simulink library "MarineRoboticsLib"  (R2022b)
settings: Solver=VariableStepAuto  StartTime=0.0  StopTime=10.0  RelTol=1e-3
undefined symbols (not defined in the file): t200_force_n, t200_pwm_n
libraries: $bdroot x13, ros2lib x4, robotcorelib x1
settings Model: Creator=dnad  LastModifiedBy=dnad

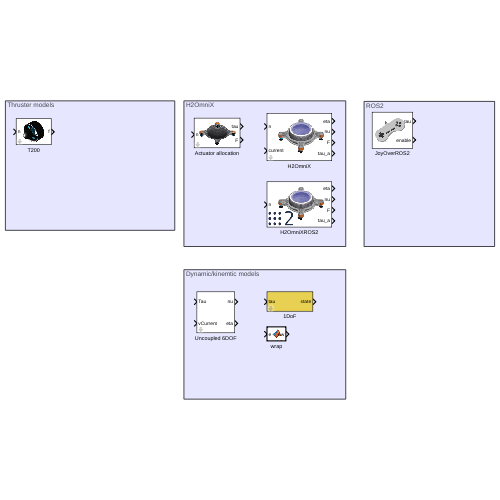
[thumbnail: Simulink's stored preview of the top-level diagram]
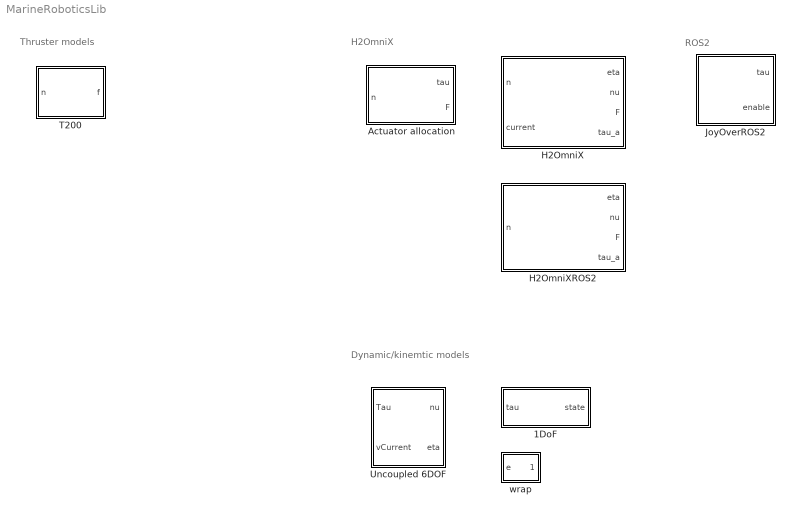
== system MarineRoboticsLib ==
  note: ROS2
  note: Dynamic/kinemtic models
  note: H2OmniX
  note: Thruster models
  1DoF : Subsystem  mask{nu0=0, alpha=0, beta=0, betaa=0}
      mask prompts: nu0 "Initial velocity"; alpha "Intertia"; beta "Linear drag"; betaa "Quadratic drag"
  Actuator allocation : Subsystem  mask(H2OmniX allocation){Tm=0, B=[0.25, 0.25, -0.25, -0.25; -0.25,  0.25, -0.25,  0.25; -0.25, 0.25, 0.25, -0.25], Keff=[1,1,1,1]}
      mask prompts: Tm "ESC time constant"; B "Thruster configuration (allocation) matrix"; Keff "Thruster efficiency (1x4 matrix)"
      mask help: The block perform normalized allocation based on thruster PWM signals and outputs the achieved generalized force and torque (tau).
      mask Display: image('$imagefile'); % Use "Edit Image" on toolstrip to change.
  H2OmniX : Subsystem  mask(H2OmniX){alpha=[2.1,2.1,0.4], beta=[0,0,0.24], betaa=[1,1,0], nu0=[0,0,0], eta0=[0,0,0]}
      mask prompts: alpha "Inertial components"; beta "Linear drag"; betaa "Quadratic drag"; nu0 "Velocities"; eta0 "Position"
      mask help: This block incorporates the H2OmniX model. It takes as input the PWM inputs for individual thrusters and sea current disturbance. It outputs the current velocity and position. For introspective purposes the individual forces applied by each thruster are output as well.
      settings: MinAlgLoopOccurrences=on
      mask DialogControl ParameterGroupVar Prompt: Dynamics
      mask DialogControl Container3 Prompt: Initial state
      mask Display: image('$imagefile'); % Use "Edit Image" on toolstrip to change.
  H2OmniXROS2 : Subsystem
      mask Display: image('$imagefile'); % Use "Edit Image" on toolstrip to change.
  JoyOverROS2 : Subsystem
      mask Display: image('$imagefile'); % Use "Edit Image" on toolstrip to change.
  T200 : Subsystem  mask(T200){Keff=1, Tm=0}
      mask prompts: Keff "Efficiency"; Tm "ESC time constant (Tm)"
      mask help: This simulink block simulates a Blue Robotics T200 thruster on 14V controlled input. The efficiancy parameter given from [0,1] additionally decreases the force output of the thruster. The ESC reaction time is the time constant of the PT1 element included in the model. Put the time constant to zero to have instantaneous response.
      mask Display: image('$imagefile'); % Use "Edit Image" on toolstrip to change.
  Uncoupled 6DOF : Subsystem  mask{nu0=[0,0,0,0,0,0], eta0=[0,0,0,0,0,0], alpha=[0,0,0,0,0,0], beta=[0,0,0,0,0,0], betaa=[0,0,0,0,0,0]}
      mask prompts: nu0 "Initial velocity"; eta0 "Initial position"; alpha "Inertia"; beta "Linear drag"; betaa "Quadratic drag"
      mask DialogControl ParameterGroupVar Prompt: Initial states
      mask DialogControl Container3 Prompt: Dynamic parameters
  wrap : MATLAB Function  TreatAsAtomicUnit=on

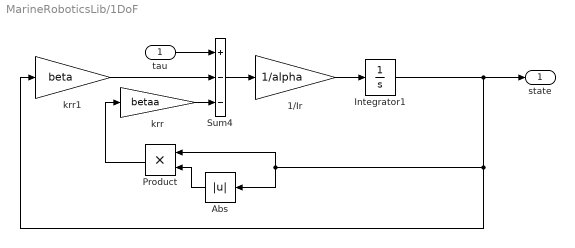
== system MarineRoboticsLib/1DoF ==
  tau : Inport
  1/Ir : Gain  Gain=1/alpha
  Abs : Abs  SaturateOnIntegerOverflow=off
  Integrator1 : Integrator  InitialCondition=nu0  UpperSaturationLimit=30*36/225*pi/180  LowerSaturationLimit=-30*36/225*pi/180
  Product : Product  RndMeth=Zero
  Sum4 : Sum  Inputs=+--
  krr : Gain  Gain=betaa
  krr1 : Gain  Gain=beta
  state : Outport
  wires:
  1/Ir/1 -> Integrator1/1
  Abs/1 -> Product/2
  Product/1 -> krr/1
  Sum4/1 -> 1/Ir/1
  krr/1 -> Sum4/3
  tau/1 -> Sum4/1
  krr1/1 -> Sum4/2
  Integrator1/1 -> krr1/1, Product/1, Abs/1, state/1

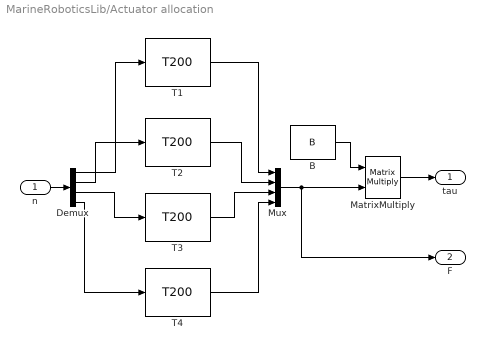
== system MarineRoboticsLib/Actuator allocation ==
  n : Inport
  B : Constant  Value=B
  Demux : Demux
  MatrixMultiply : Product  Multiplication=Matrix(*)
  Mux : Mux
  T1 : $bdroot/T200  Keff=Keff(1)  Tm=Tm
  T2 : $bdroot/T200  Keff=Keff(2)  Tm=Tm
  T3 : $bdroot/T200  Keff=Keff(3)  Tm=Tm
  T4 : $bdroot/T200  Keff=Keff(4)  Tm=Tm
  tau : Outport
  F : Outport  Port=2
  wires:
  T2/1 -> Mux/2
  Demux/2 -> T2/1
  T1/1 -> Mux/1
  T4/1 -> Mux/4
  T3/1 -> Mux/3
  Mux/1 -> F/1, MatrixMultiply/2
  Demux/1 -> T1/1
  Demux/4 -> T4/1
  Demux/3 -> T3/1
  B/1 -> MatrixMultiply/1
  n/1 -> Demux/1
  MatrixMultiply/1 -> tau/1

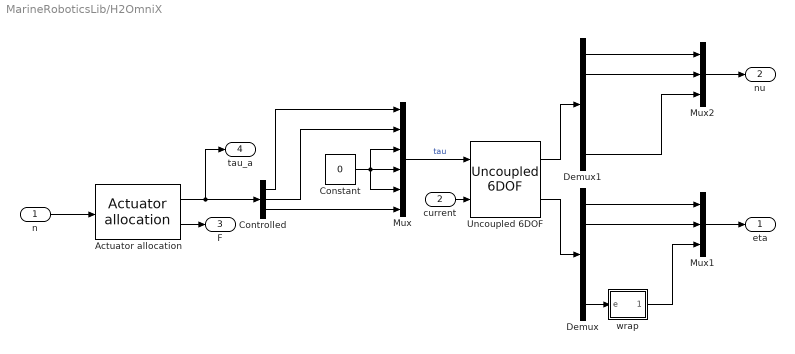
== system MarineRoboticsLib/H2OmniX ==
  n : Inport
  current : Inport  Port=2
  Actuator allocation : $bdroot/Actuator allocation  Tm=0  B="[0.25, 0.25, -0.25, -0.25; -0.25,  0.25, -0.25,  0.25; -0.25, 0.25, 0.25, -0.25]"  Keff=[1,1,1,1]
  Constant : Constant  Value=0
  Controlled : Demux  Outputs=3
  Demux : Demux  Outputs=6
  Demux1 : Demux  Outputs=6
  Mux : Mux  Inputs=6
  Mux1 : Mux  Inputs=3
  Mux2 : Mux  Inputs=3
  Uncoupled 6DOF : $bdroot/Uncoupled 6DOF  nu0=[nu0(1) nu0(2) 0 0 0 nu0(3)]  eta0=[eta0(1) eta0(2) 0 0 0 eta0(3)]  alpha=[alpha(1) alpha(2) 1000 1000 1000 alpha(3)]  beta=[beta(1) beta(2) 0 0 0 beta(3)]  betaa=[betaa(1) betaa(2) 0 0 0 betaa(3)]
  wrap : MATLAB Function  TreatAsAtomicUnit=on
  eta : Outport
  nu : Outport  Port=2
  F : Outport  Port=3
  tau_a : Outport  Port=4
  wires:
  n/1 -> Actuator allocation/1
  Mux/1 -> Uncoupled 6DOF/1  "tau"
  Actuator allocation/1 -> tau_a/1, Controlled/1
  Controlled/1 -> Mux/1
  Controlled/2 -> Mux/2
  Controlled/3 -> Mux/6
  current/1 -> Uncoupled 6DOF/2
  Actuator allocation/2 -> F/1
  Constant/1 -> Mux/5, Mux/4, Mux/3
  Uncoupled 6DOF/2 -> Demux/1
  Mux1/1 -> eta/1
  Demux/1 -> Mux1/1
  Demux/2 -> Mux1/2
  Demux/6 -> wrap/1(e)
  wrap/1(ew) -> Mux1/3
  Uncoupled 6DOF/1 -> Demux1/1
  Mux2/1 -> nu/1
  Demux1/1 -> Mux2/1
  Demux1/2 -> Mux2/2
  Demux1/6 -> Mux2/3

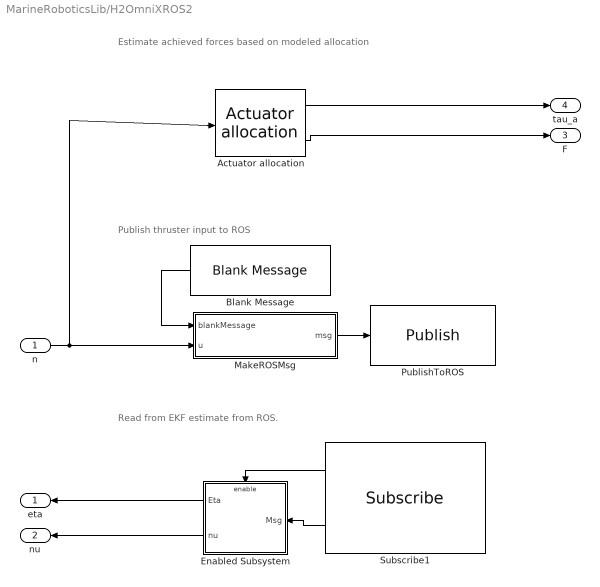
== system MarineRoboticsLib/H2OmniXROS2 ==
  note: Read from EKF estimate from ROS.
  note: Publish thruster input to ROS
  note: Estimate achieved forces based on modeled allocation
  n : Inport
  Actuator allocation : $bdroot/Actuator allocation  Tm=0  B="[0.25, 0.25, -0.25, -0.25; -0.25,  0.25, -0.25,  0.25; -0.25, 0.25, 0.25, -0.25]"  Keff=[1,1,1,1]
  Blank Message : ros2lib/Blank Message  messageClass=Message  entityType=std_msgs/Float32MultiArray  messageType=std_msgs/Float32MultiArray  SampleTime=0.05
  Enabled Subsystem : Subsystem  TreatAsAtomicUnit=on
  MakeROSMsg : MATLAB Function  TreatAsAtomicUnit=on  SystemSampleTime=0.05
  PublishToROS : ros2lib/Publish  topicSource=Specify your own  topic=/h2omnix/pwm_out  messageType=std_msgs/Float32MultiArray  QOSHistory=Keep last  QOSDepth=10  QOSReliability=Reliable  QOSDurability=Volatile
  Subscribe1 : ros2lib/Subscribe  topicSource=Specify your own  topic=/h2omnix/odometry/filtered  messageType=nav_msgs/Odometry  sampleTime=0.01  QOSHistory=Keep last  QOSDepth=1  QOSReliability=Reliable  QOSDurability=Volatile
  eta : Outport
  nu : Outport  Port=2
  F : Outport  Port=3
  tau_a : Outport  Port=4
  wires:
  MakeROSMsg/1(msg) -> PublishToROS/1
  Subscribe1/2 -> Enabled Subsystem/1(Msg)
  Subscribe1/1 -> Enabled Subsystem/Enable
  Enabled Subsystem/1(Eta) -> eta/1
  Blank Message/1 -> MakeROSMsg/1(blankMessage)
  n/1 -> Actuator allocation/1, MakeROSMsg/2(u)
  Enabled Subsystem/2(nu) -> nu/1
  Actuator allocation/2 -> F/1
  Actuator allocation/1 -> tau_a/1

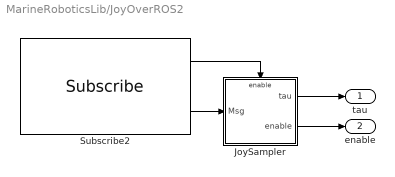
== system MarineRoboticsLib/JoyOverROS2 ==
  JoySampler : Subsystem  TreatAsAtomicUnit=on
  Subscribe2 : ros2lib/Subscribe  topicSource=Specify your own  topic=/h2omnix/joy  messageType=sensor_msgs/Joy  sampleTime=0.01  QOSHistory=Keep last  QOSDepth=1  QOSReliability=Reliable  QOSDurability=Volatile
  tau : Outport
  enable : Outport  Port=2
  wires:
  Subscribe2/2 -> JoySampler/1(Msg)
  Subscribe2/1 -> JoySampler/Enable
  JoySampler/2(enable) -> enable/1
  JoySampler/1(tau) -> tau/1

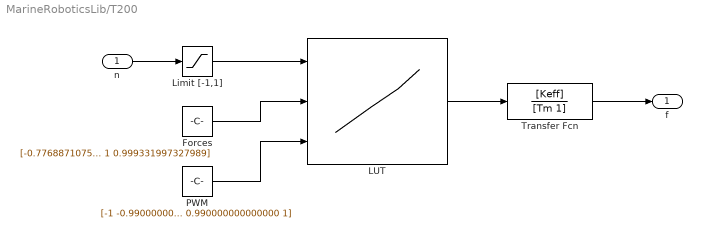
== system MarineRoboticsLib/T200 ==
  n : Inport
  Forces : Constant  Value=|
      | [-0.776887107548430
      | -0.772545090180361
      | -0.771543086172345
      | -0.762525050100200
      | -0.751503006012024
      | -0.741482965931864
      | -0.727454909819639
      | -0.717434869739479
      | -0.704408817635270
      | -0.693386773547094
      | -0.684368737474950
      | -0.675350701402806
      | -0.663326653306613
      | -0.649298597194389
      | -0.637274549098196
      | -0.629258517034068
      | -0.614228456913828
      | -0.610220440881764
      | -0.594188376753507
      | -0.584168336673347
      | -0.573146292585170
      | -0.558116232464930
      | -0.550100200400802
      | -0.542084168336673
      | -0.532064128256513
      | -0.519038076152305
      | -0.516032064128256
      | -0.498997995991984
      | -0.486973947895792
      | -0.480961923847695
      | -0.467935871743487
      | -0.453907815631262
      | -0.447895791583166
      | -0.438877755511022
      | -0.421843687374750
      | -0.417835671342685
      | -0.401803607214429
      | -0.389779559118237
      | -0.379759519038076
      | -0.371743486973948
      | -0.360721442885772
      | -0.348697394789579
      | -0.345691382765531
      | -0.335671342685371
      | -0.326653306613226
      | -0.318637274549098
      | -0.309619238476954
      | -0.302605210420842
      | -0.292585170340681
      | -0.283567134268537
      | -0.273547094188377
      | -0.263527054108217
      | -0.257515030060120
      | -0.248496993987976
      | -0.240480961923848
      | -0.232464929859719
      | -0.224448897795591
      | -0.217434869739479
      | -0.210420841683367
      | -0.202404809619238
      | -0.195390781563126
      | -0.187374749498998
      | -0.178356713426854
      | -0.169338677354709
      | -0.163326653306613
      | -0.155310621242485
      | -0.150300601202405
      | -0.143286573146293
      | -0.137274549098196
      | -0.129258517034068
      | -0.121242484969940
      | -0.114228456913828
      | -0.108216432865731
      | -0.102204408817635
      | -0.0941883767535070
      | -0.0881763527054108
      | -0.0821643286573146
      | -0.0771543086172345
      | -0.0701402805611222
      | -0.0631262525050100
      | -0.0571142284569138
      | -0.0521042084168337
      | -0.0460921843687375
      | -0.0410821643286573
      | -0.0360721442885772
      | -0.0320641282565130
      | -0.0270541082164329
      | -0.0220440881763527
      | -0.0180360721442886
      | -0.0150300601202405
      | -0.0100200400801603
      | -0.00701402805611223
      | 0
      | 0
      | 0
      | 0
      | 0
      | 0
      | 0
      | 0
      | 0
      | 0
      | 0
      | 0
      | 0
      | 0
      | 0
      | 0
      | 0
      | 0.0100200400801603
      | 0.0140280561122245
      | 0.0180360721442886
      | 0.0220440881763527
      | 0.0270541082164329
      | 0.0320641282565130
      | 0.0390781563126253
      | 0.0440881763527054
      | 0.0501002004008016
      | 0.0581162324649299
      | 0.0641282565130261
      | 0.0721442885771543
      | 0.0801603206412826
      | 0.0871743486973948
      | 0.0941883767535070
      | 0.102204408817635
      | 0.110220440881764
      | 0.117234468937876
      | 0.127254509018036
      | 0.137274549098196
      | 0.142284569138277
      | 0.152304609218437
      | 0.160320641282565
      | 0.169338677354709
      | 0.182364729458918
      | 0.187374749498998
      | 0.196392785571142
      | 0.203406813627254
      | 0.213426853707415
      | 0.220440881763527
      | 0.232464929859719
      | 0.241482965931864
      | 0.252505010020040
      | 0.265531062124249
      | 0.272545090180361
      | 0.282565130260521
      | 0.292585170340681
      | 0.301603206412826
      | 0.310621242484970
      | 0.322645290581162
      | 0.333667334669339
      | 0.342685370741483
      | 0.354709418837675
      | 0.364729458917836
      | 0.377755511022044
      | 0.388777555110220
      | 0.400801603206413
      | 0.408817635270541
      | 0.421843687374750
      | 0.433867735470942
      | 0.442885771543086
      | 0.460921843687375
      | 0.467935871743487
      | 0.476953907815631
      | 0.495991983967936
      | 0.501002004008016
      | 0.517034068136273
      | 0.536072144288577
      | 0.553106212424850
      | 0.566132264529058
      | 0.582164328657315
      | 0.587174348697395
      | 0.609218436873748
      | 0.614228456913828
      | 0.636272545090180
      | 0.648296593186373
      | 0.661322645290581
      | 0.673346693386774
      | 0.691382765531062
      | 0.704408817635271
      | 0.714428857715431
      | 0.734468937875751
      | 0.742484969939880
      | 0.755511022044088
      | 0.771543086172345
      | 0.787575150300601
      | 0.800601202404810
      | 0.814629258517034
      | 0.832665330661323
      | 0.847695390781563
      | 0.866733466933868
      | 0.879759519038076
      | 0.889779559118237
      | 0.907815631262525
      | 0.917835671342685
      | 0.930861723446894
      | 0.950901803607214
      | 0.967935871743487
      | 0.976953907815631
      | 0.995991983967936
      | 1
      | 0.999331997327989]
  LUT : Lookup_n-D  NumberOfTableDimensions=1  BreakpointsForDimension1Source=Input port  BreakpointsForDimension1=t200_pwm_n  TableSource=Input port  Table=t200_force_n  InternalRulePriority=Speed  RndMeth=Simplest
      settings: InputPortMap=u0,p221,p5
  Limit [-1,1] : Saturate  UpperLimit=1  LowerLimit=-1
  PWM : Constant  Value=|
      | [-1
      | -0.990000000000000
      | -0.980000000000000
      | -0.970000000000000
      | -0.960000000000000
      | -0.950000000000000
      | -0.940000000000000
      | -0.930000000000000
      | -0.920000000000000
      | -0.910000000000000
      | -0.900000000000000
      | -0.890000000000000
      | -0.880000000000000
      | -0.870000000000000
      | -0.860000000000000
      | -0.850000000000000
      | -0.840000000000000
      | -0.830000000000000
      | -0.820000000000000
      | -0.810000000000000
      | -0.800000000000000
      | -0.790000000000000
      | -0.780000000000000
      | -0.770000000000000
      | -0.760000000000000
      | -0.750000000000000
      | -0.740000000000000
      | -0.730000000000000
      | -0.720000000000000
      | -0.710000000000000
      | -0.700000000000000
      | -0.690000000000000
      | -0.680000000000000
      | -0.670000000000000
      | -0.660000000000000
      | -0.650000000000000
      | -0.640000000000000
      | -0.630000000000000
      | -0.620000000000000
      | -0.610000000000000
      | -0.600000000000000
      | -0.590000000000000
      | -0.580000000000000
      | -0.570000000000000
      | -0.560000000000000
      | -0.550000000000000
      | -0.540000000000000
      | -0.530000000000000
      | -0.520000000000000
      | -0.510000000000000
      | -0.500000000000000
      | -0.490000000000000
      | -0.480000000000000
      | -0.470000000000000
      | -0.460000000000000
      | -0.450000000000000
      | -0.440000000000000
      | -0.430000000000000
      | -0.420000000000000
      | -0.410000000000000
      | -0.400000000000000
      | -0.390000000000000
      | -0.380000000000000
      | -0.370000000000000
      | -0.360000000000000
      | -0.350000000000000
      | -0.340000000000000
      | -0.330000000000000
      | -0.320000000000000
      | -0.310000000000000
      | -0.300000000000000
      | -0.290000000000000
      | -0.280000000000000
      | -0.270000000000000
      | -0.260000000000000
      | -0.250000000000000
      | -0.240000000000000
      | -0.230000000000000
      | -0.220000000000000
      | -0.210000000000000
      | -0.200000000000000
      | -0.190000000000000
      | -0.180000000000000
      | -0.170000000000000
      | -0.160000000000000
      | -0.150000000000000
      | -0.140000000000000
      | -0.130000000000000
      | -0.120000000000000
      | -0.110000000000000
      | -0.100000000000000
      | -0.0900000000000000
      | -0.0800000000000000
      | -0.0700000000000000
      | -0.0600000000000000
      | -0.0500000000000000
      | -0.0400000000000000
      | -0.0300000000000000
      | -0.0200000000000000
      | -0.0100000000000000
      | 0
      | 0.0100000000000000
      | 0.0200000000000000
      | 0.0300000000000000
      | 0.0400000000000000
      | 0.0500000000000000
      | 0.0600000000000000
      | 0.0700000000000000
      | 0.0800000000000000
      | 0.0900000000000000
      | 0.100000000000000
      | 0.110000000000000
      | 0.120000000000000
      | 0.130000000000000
      | 0.140000000000000
      | 0.150000000000000
      | 0.160000000000000
      | 0.170000000000000
      | 0.180000000000000
      | 0.190000000000000
      | 0.200000000000000
      | 0.210000000000000
      | 0.220000000000000
      | 0.230000000000000
      | 0.240000000000000
      | 0.250000000000000
      | 0.260000000000000
      | 0.270000000000000
      | 0.280000000000000
      | 0.290000000000000
      | 0.300000000000000
      | 0.310000000000000
      | 0.320000000000000
      | 0.330000000000000
      | 0.340000000000000
      | 0.350000000000000
      | 0.360000000000000
      | 0.370000000000000
      | 0.380000000000000
      | 0.390000000000000
      | 0.400000000000000
      | 0.410000000000000
      | 0.420000000000000
      | 0.430000000000000
      | 0.440000000000000
      | 0.450000000000000
      | 0.460000000000000
      | 0.470000000000000
      | 0.480000000000000
      | 0.490000000000000
      | 0.500000000000000
      | 0.510000000000000
      | 0.520000000000000
      | 0.530000000000000
      | 0.540000000000000
      | 0.550000000000000
      | 0.560000000000000
      | 0.570000000000000
      | 0.580000000000000
      | 0.590000000000000
      | 0.600000000000000
      | 0.610000000000000
      | 0.620000000000000
      | 0.630000000000000
      | 0.640000000000000
      | 0.650000000000000
      | 0.660000000000000
      | 0.670000000000000
      | 0.680000000000000
      | 0.690000000000000
      | 0.700000000000000
      | 0.710000000000000
      | 0.720000000000000
      | 0.730000000000000
      | 0.740000000000000
      | 0.750000000000000
      | 0.760000000000000
      | 0.770000000000000
      | 0.780000000000000
      | 0.790000000000000
      | 0.800000000000000
      | 0.810000000000000
      | 0.820000000000000
      | 0.830000000000000
      | 0.840000000000000
      | 0.850000000000000
      | 0.860000000000000
      | 0.870000000000000
      | 0.880000000000000
      | 0.890000000000000
      | 0.900000000000000
      | 0.910000000000000
      | 0.920000000000000
      | 0.930000000000000
      | 0.940000000000000
      | 0.950000000000000
      | 0.960000000000000
      | 0.970000000000000
      | 0.980000000000000
      | 0.990000000000000
      | 1]
  Transfer Fcn : TransferFcn  Numerator=[Keff]  Denominator=[Tm 1]
  f : Outport
  wires:
  Limit [-1,1]/1 -> LUT/1
  LUT/1 -> Transfer Fcn/1
  n/1 -> Limit [-1,1]/1
  Transfer Fcn/1 -> f/1
  Forces/1 -> LUT/2
  PWM/1 -> LUT/3

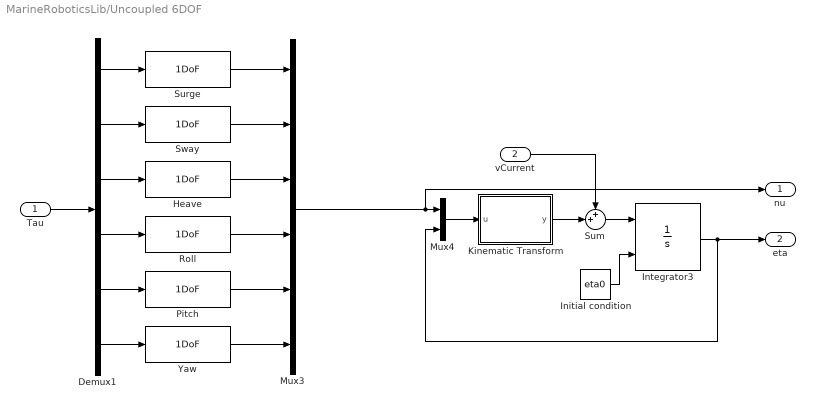
== system MarineRoboticsLib/Uncoupled 6DOF ==
  Tau : Inport
  vCurrent : Inport  Port=2
  Demux1 : Demux  Outputs=6
  Heave : $bdroot/1DoF  nu0=nu0(3)  alpha=alpha(3)  beta=beta(3)  betaa=betaa(3)
  Initial condition : Constant  Value=eta0
  Integrator3 : Integrator  InitialConditionSource=external
  Kinematic Transform : MATLAB Function  TreatAsAtomicUnit=on
  Mux3 : Mux  Inputs=6
  Mux4 : Mux  Inputs=2
  Pitch : $bdroot/1DoF  nu0=nu0(5)  alpha=alpha(5)  beta=beta(5)  betaa=betaa(5)
  Roll : $bdroot/1DoF  nu0=nu0(4)  alpha=alpha(4)  beta=beta(4)  betaa=betaa(4)
  Sum : Sum  Inputs=++|
  Surge : $bdroot/1DoF  nu0=nu0(1)  alpha=alpha(1)  beta=beta(1)  betaa=betaa(1)
  Sway : $bdroot/1DoF  nu0=nu0(2)  alpha=alpha(2)  beta=beta(2)  betaa=betaa(2)
  Yaw : $bdroot/1DoF  nu0=nu0(6)  alpha=alpha(6)  beta=beta(6)  betaa=betaa(6)
  nu : Outport
  eta : Outport  Port=2
  wires:
  Tau/1 -> Demux1/1
  Demux1/1 -> Surge/1
  Demux1/3 -> Heave/1
  Demux1/6 -> Yaw/1
  Demux1/5 -> Pitch/1
  Demux1/4 -> Roll/1
  Demux1/2 -> Sway/1
  Mux4/1 -> Kinematic Transform/1(u)
  Integrator3/1 -> eta/1, Mux4/2
  Surge/1 -> Mux3/1
  Sway/1 -> Mux3/2
  Heave/1 -> Mux3/3
  Roll/1 -> Mux3/4
  Pitch/1 -> Mux3/5
  Yaw/1 -> Mux3/6
  Initial condition/1 -> Integrator3/2
  Kinematic Transform/1(y) -> Sum/2
  Sum/1 -> Integrator3/1
  vCurrent/1 -> Sum/1
  Mux3/1 -> nu/1, Mux4/1

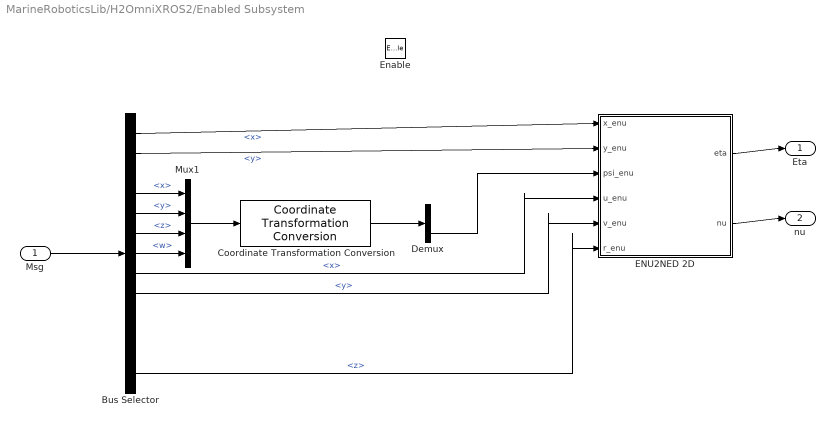
== system MarineRoboticsLib/H2OmniXROS2/Enabled Subsystem ==
  Msg : Inport
  Enable : EnablePort
  Bus Selector : BusSelector  OutputSignals=pose.pose.position.x,pose.pose.position.y,pose.pose.position.z,pose.pose.orientation.x,pose.pose.orientation.y,pose.pose.orientation.z,pose.pose.orientation.w,twist.twist.linear.x,twist.twist.linear.y,twist.twist.linear.z,twist.twist.angular.x,twist.twist.angular.y,twist.twist.angular.z
  Coordinate Transformation Conversion : robotcorelib/Coordinate Transformation Conversion  InputRepresentation=Quaternion  InputEulerSequence=ZYX  ShowTrVecInputPort=on  OutputRepresentation=Euler Angles  OutputEulerSequence=ZYX  ShowTrVecOutputPort=on  SimulateUsing=Interpreted execution
      settings: LibrarySourceBlock=roslib/Utilities/Coordinate Transformation Conversion
  Demux : Demux  Outputs=3
  ENU2NED 2D : MATLAB Function  TreatAsAtomicUnit=on
  Mux1 : Mux
  Eta : Outport
  nu : Outport  Port=2
  wires:
  Msg/1 -> Bus Selector/1
  Bus Selector/4 -> Mux1/1  "<x>"
  Bus Selector/5 -> Mux1/2  "<y>"
  Bus Selector/6 -> Mux1/3  "<z>"
  Bus Selector/7 -> Mux1/4  "<w>"
  Mux1/1 -> Coordinate Transformation Conversion/1
  Bus Selector/2 -> ENU2NED 2D/2(y_enu)  "<y>"
  Bus Selector/1 -> ENU2NED 2D/1(x_enu)  "<x>"
  Coordinate Transformation Conversion/1 -> Demux/1
  Bus Selector/8 -> ENU2NED 2D/4(u_enu)  "<x>"
  Bus Selector/9 -> ENU2NED 2D/5(v_enu)  "<y>"
  Bus Selector/13 -> ENU2NED 2D/6(r_enu)  "<z>"
  ENU2NED 2D/1(eta) -> Eta/1
  ENU2NED 2D/2(nu) -> nu/1
  Demux/3 -> ENU2NED 2D/3(psi_enu)

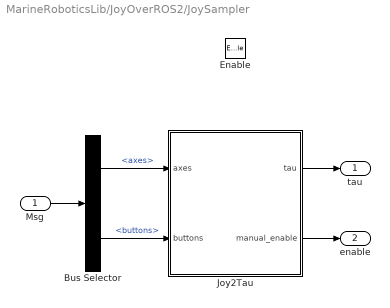
== system MarineRoboticsLib/JoyOverROS2/JoySampler ==
  Msg : Inport
  Enable : EnablePort
  Bus Selector : BusSelector  OutputSignals=axes,buttons
  Joy2Tau : MATLAB Function  TreatAsAtomicUnit=on
  tau : Outport
  enable : Outport  Port=2
  wires:
  Msg/1 -> Bus Selector/1
  Joy2Tau/1(tau) -> tau/1
  Joy2Tau/2(manual_enable) -> enable/1
  Bus Selector/2 -> Joy2Tau/2(buttons)  "<buttons>"
  Bus Selector/1 -> Joy2Tau/1(axes)  "<axes>"

== matlab function MarineRoboticsLib/H2OmniXROS2/MakeROSMsg ==
  data: blankMessage input; u input; msg output Bus: SL_Bus_std_msgs_Float32MultiArray
function msg  = assign_bus(blankMessage,u)

% blank message input
msg = blankMessage;

% assign pwm values into data field
msg.data(1:numel(u)) = reshape(u,[],1);

% all other fields must be assigned to complete the message
msg.data_SL_Info.CurrentLength = uint32(numel(u));
msg.layout.dim(1).size = uint32(size(u,1));
msg.layout.dim(2).size = uint32(size(u,2));
msg.layout.dim(1).stride = uint32(numel(u));
msg.layout.dim(2).stride = uint32(prod(size(u,2)));

== matlab function MarineRoboticsLib/Uncoupled 6DOF/Kinematic Transform ==
  data: u input; y output
function y = fcn(u)
%#codegen
if (length(u)<12) 
    y = zeros(12,1);
    return;
end

input = u;
% Read inputs
u = input(1,1);
v = input(2,1);
w = input(3,1);
p = input(4,1);
q = input(5,1);
r = input(6,1);

%x = input(7,1);
%y = input(8,1);
%z = input(9,1);
phi = input(10,1);
theta = input(11,1);
Psi = input(12,1);

DOF6 = 1; % Select degrees of freedom

tmp1 = []; tmp2 = [];

if DOF6 == 1
    
    % Rotation matrix
    R_x_phi = [1 0 0; 0 cos(phi) sin(phi); 0 -sin(phi) cos(phi)];
    R_y_theta = [cos(theta) 0 -sin(theta); 0 1 0; sin(theta) 0 cos(theta)];% Provjeri matrice
    R_z_psi = [cos(Psi) sin(Psi) 0; -sin(Psi) cos(Psi) 0; 0 0 1];
    
    % Linear velocity transform
    J1 = R_z_psi.'*R_y_theta.'*R_x_phi.';
    
    % Angular velocity transform    
    tmp1 = R_x_phi(:,2);
    tmp1 = [0 0 0; tmp1.'; 0 0 0].';
    
    tmp2 = R_x_phi*R_y_theta;
    tmp2 = tmp2(:,3);
    tmp2 = [0 0 0; 0 0 0; tmp2.'].';
    
    J2 = inv(diag([1 0 0])+tmp1+tmp2);
    
elseif DOF6 == 0
    
    % Rotation matrix
    R_x_phi = eye(3);
    R_y_theta = eye(3);
    R_z_psi = [cos(Psi) sin(Psi) 0; -sin(Psi) cos(Psi) 0; 0 0 1]; % Provjeri matrice
    
    % Linear velocity transform
    J1 = R_z_psi.'*R_y_theta.'*R_x_phi.';
    
    % Angular velocity transform 
    tmp1 = R_x_phi(:,2);
    tmp1 = [0 0 0; tmp1.'; 0 0 0].';
    
    tmp2 = R_x_phi*R_y_theta;
    tmp2 = tmp2(:,3);
    tmp2 = [0 0 0; 0 0 0; tmp2.'].';
    
    J2 = inv(diag([1 0 0])+tmp1+tmp2);
    
end

eta1 = J1*[u v w].';
eta2 = J2*[p q r].';


y = [eta1.' eta2.'].';

== matlab function MarineRoboticsLib/H2OmniX/wrap ==
  data: e input; ew output
function ew = wrap(e)

ew = mod(e, 2*pi);

if ew > pi
   ew = -2*pi + ew;
elseif ew <= -pi 
   ew = 2*pi + ew;
end

== matlab function MarineRoboticsLib/wrap ==
  data: e input; ew output
function ew = wrap(e)

ew = mod(e, 2*pi);

if ew > pi
   ew = -2*pi + ew;
elseif ew <= -pi 
   ew = 2*pi + ew;
end

== matlab function MarineRoboticsLib/H2OmniXROS2/Enabled Subsystem/ENU2NED 2D ==
  data: x_enu input; eta output; y_enu input; psi_enu input; u_enu input; v_enu input; r_enu input; nu output
function [eta, nu] = enu2ned2d(x_enu,y_enu,psi_enu,u_enu,v_enu,r_enu)
% Just do coordinate swap
eta = [y_enu; x_enu; pi/2-psi_enu];
nu = [v_enu; x_enu; -r_enu;];

== matlab function MarineRoboticsLib/JoyOverROS2/JoySampler/Joy2Tau ==
  data: axes input; tau output; buttons input; manual_enable output
function [tau, manual_enable] = joy2tau(axes, buttons)

% JUST X,Y,N for now
if length(axes) > 3
    tau = [axes(2); -axes(1); -axes(3)];
end
manual_enable = buttons(1);
